simulink model "AAS"  (R2022b)
settings: Solver=ode4  StartTime=0.0  StopTime=inf  FixedStep=0.01  RelTol=1e-3  EnableMultiTasking=on
libraries: fuzblock x1
settings Model: Creator=marwa  LastModifiedBy=marwa
settings SolverCC: AlgebraicLoopSolver=TrustRegion  AutoInsertRateTranBlk=on
settings DataIOCC: LimitDataPoints=on
settings OptimizationCC: LifeSpan=inf
settings DebuggingCC: UnconnectedInputMsg=warning  UnconnectedOutputMsg=warning  UnconnectedLineMsg=warning  AllowSymbolicDim=off  SFUnexpectedBacktrackingDiag=warning  SFNoUnconditionalDefaultTransitionDiag=warning  SFExecutionAtInitializationDiag=none  ArithmeticOperatorsInVariantConditions=warning
settings ModelReferenceCC: EnableRefExpFcnMdlSchedulingChecks=on
settings SFSimCC: SimUseLocalCustomCode=off  CustomCodeUndefinedFunction=UseInterfaceOnly
settings RTWCC: RTWUseLocalCustomCode=off  DLArmComputeVersion=19.05
settings CodeAppCC: StateflowObjectComments=on
settings GRTTargetCC: TargetLangStandard=C89/C90 (ANSI)
settings ConfigComp: CovMetricSettings=dw  CovSaveCumulativeToWorkspaceVar=on  CovSaveSingleToWorkspaceVar=on  CovExternalEMLEnable=off  CovSFcnEnable=off

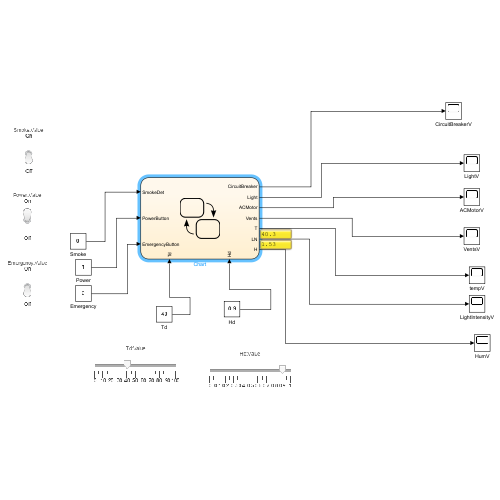
[thumbnail: Simulink's stored preview of the top-level diagram]
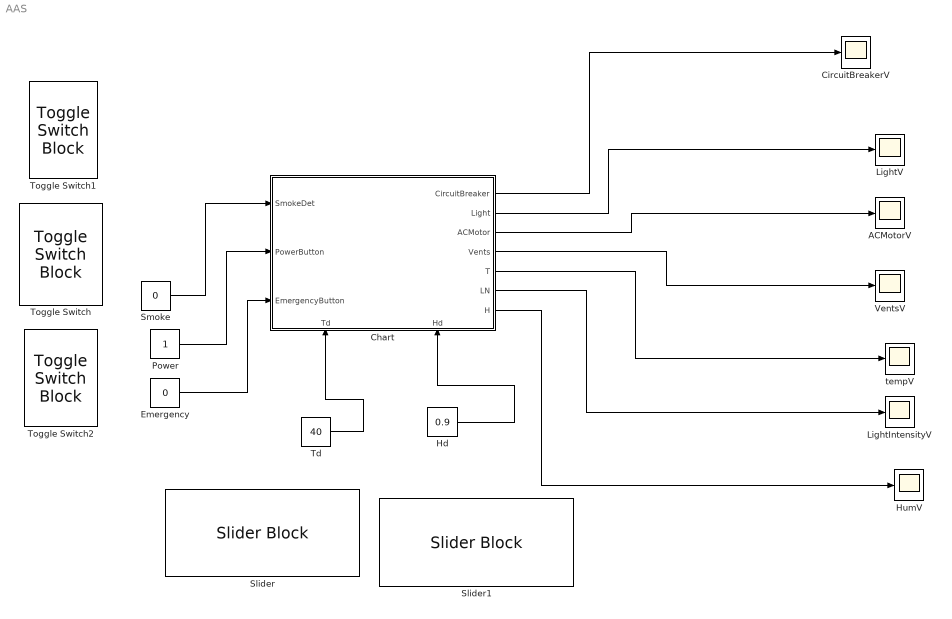
== system AAS ==
  ACMotorV : Scope
  Chart : Stateflow chart  TreatAsAtomicUnit=on
      settings: PortSchema="{\"entries\":[{\"content\":{\"sides\":[{\"content\":{\"connectorIds\":[\"In1\",\"In2\",\"In3\"]},\"type\":\"ConnectorPlacement.EquallySpacedRectSide\",\"uuid\":\"5cb868e6-5551-4fae-9f9a-b14f0c4a41d3\"},{\"content\":{\"connectorIds\":[\"Out1\",\"Out2\",\"Out3\",\"Out4\",\"Out6\",\"Out5\",\"Out7\"],\"side\":\"RIGHT\"},\"type\":\"ConnectorPlacement.EquallySpacedRectSide\",\"uuid\":\"822cf98d-9f25-4796-a860-f61431df4421\"},{\"content\":{\"connectorIds\":[],\"side\":\"TOP\"},\"type\":\"ConnectorPlacement.EquallySpacedRectSide\",\"uuid\":\"1de60880-a042-4c2a-a744-54787d460a6d\"},{\"content\":{\"connectorIds\":[\"In4\",\"In5\"],\"side\":\"BOTTOM\"},\"type\":\"ConnectorPlacement.EquallySpacedRectSide\",\"uuid\":\"160f7fd3-c7f7-4859-8f15-e416a90d14eb\"}]},\"type\":\"ConnectorPlacement.EquallySpacedConnector\",\"uuid\":\"910f53eb-049d-4d7c-afd0-ebd92eccdf07\"}],\"packageUris\":[\"http://schema.mathworks.com/mf0/Connector/R2020b\"],\"version\":\"1.0\"}"
  CircuitBreakerV : Scope
  Emergency : Constant  Value=0
  Hd : Constant  Value=0.9
  HumV : Scope
  LightIntensityV : Scope
  LightV : Scope
  Power : Constant
  Slider : SliderBlock
  Slider1 : SliderBlock  ScaleMax=1
  Smoke : Constant  Value=0
  Td : Constant  Value=40
  Toggle Switch : ToggleSwitchBlock
      settings: Values={{'Off', 'On'}, [0 1]}
  Toggle Switch1 : ToggleSwitchBlock
      settings: Values={{'Off', 'On'}, [0 1]}
  Toggle Switch2 : ToggleSwitchBlock
      settings: Values={{'Off', 'On'}, [0 1]}
  VentsV : Scope
  tempV : Scope
  wires:
  Power/1 -> Chart/2(PowerButton)
  Smoke/1 -> Chart/1(SmokeDet)
  Emergency/1 -> Chart/3(EmergencyButton)
  Chart/1(CircuitBreaker) -> CircuitBreakerV/1
  Chart/2(Light) -> LightV/1
  Chart/3(ACMotor) -> ACMotorV/1
  Chart/6(T) -> tempV/1
  Chart/4(Vents) -> VentsV/1
  Chart/5(LN) -> LightIntensityV/1
  Chart/7(H) -> HumV/1
  Td/1 -> Chart/4(Td)
  Hd/1 -> Chart/5(Hd)

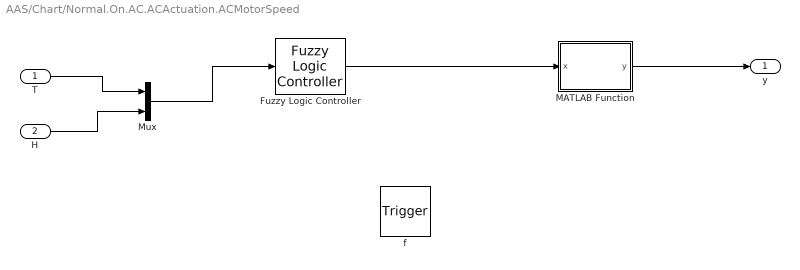
== system AAS/Chart/Normal.On.AC.ACActuation.ACMotorSpeed ==
  T : Inport  OutDataTypeStr=double  PortDimensions=1
  H : Inport  Port=2  OutDataTypeStr=double  PortDimensions=1
  f : TriggerPort  TriggerType=function-call  VariantControl=(inherit)
      settings: CopyFcn=Stateflow.SLINSF.SimulinkMan.removeBlockPreDeleteFcn  PreDeleteFcn=Stateflow.SLINSF.SimulinkMan.unsafePredeleteFcn
  Fuzzy Logic Controller : fuzblock/Fuzzy Logic  Controller  FIS=FuzzyAdvanced  OutputSampleNumber=101  DataType=double  FuzzifiedInputs=off  RuleFiringStrengths=off  RuleOutputs=off  AggregatedOutputs=off  SimulateUsing=Interpreted execution  OutOfRangeInputValueMessage=warning  NoRuleFiredMessage=warning  EmptyOutputFuzzySetMessage=warning
  MATLAB Function : MATLAB Function  TreatAsAtomicUnit=on
  Mux : Mux  Inputs=2
  y : Outport
  wires:
  T/1 -> Mux/1
  H/1 -> Mux/2
  MATLAB Function/1(y) -> y/1
  Fuzzy Logic Controller/1 -> MATLAB Function/1(x)
  Mux/1 -> Fuzzy Logic Controller/1

== matlab function AAS/Chart/Normal.On.AC.ACActuation.ACMotorSpeed/MATLAB Function ==
  data: x input; y output
function y = fcn(x)
y = 1725*(1-x)+1725;

== stateflow chart AAS/Chart ==
  settings: updateMethod=CONTINUOUS
  state Normal
    entry:
    Vents = 0;
    CircuitBreaker = 0;
    state On
      state Light [parallel]
        settings: executionOrder=2
        state LightSensing [parallel]
          settings: executionOrder=2
          state Day
            du:
            LN_dot = LN /100;
          state Night
            du:
            LN_dot = -LN/100;
          (default) -> Night
          Day -> Night : [LN > 100]
          Night -> Day : [LN < 1]
        state LightActuation [parallel]
          settings: executionOrder=1
          (history)
          state Zero
            entry:
            Light = 0;
            %0 dark
            %100 light
          state Quarter
            entry:
            Light = 25;
          state Half
            entry:
            Light = 50;
          state Maximum
            entry:
            Light = 100;
          state ThreeQuarter
            entry:
            Light = 75;
          (default) -> Zero
          Quarter -> Half [order 1] : [LN < 75]
          Zero -> Quarter : [LN < 100]
          Quarter -> Zero [order 2] : [LN >= 100]
          Half -> Quarter [order 2] : [LN >= 75]
          ThreeQuarter -> Half [order 2] : [LN >= 50]
          Half -> ThreeQuarter [order 1] : [LN < 50]
          ThreeQuarter -> Maximum [order 1] : [LN < 25]
          Maximum -> ThreeQuarter : [LN >= 25]
      state AC [parallel]
        settings: executionOrder=1
        state TempSensing [parallel]
          settings: executionOrder=1
          state Below
            du:
            T_dot = -T;
          state Over
            du:
            T_dot = 100 - T;
          state Regulated
            du:
            T_dot = 0;
          (default) -> Normal.On.AC.TempSensing.Below
          Normal.On.AC.TempSensing.Over -> Normal.On.AC.TempSensing.Below [order 1] : [int_num(T) > int_num(Td)]
          Normal.On.AC.TempSensing.Below -> Normal.On.AC.TempSensing.Over [order 1] : [int_num(T) < int_num(Td)]
          Normal.On.AC.TempSensing.Below -> Normal.On.AC.TempSensing.Regulated [order 2] : [(int_num(T) - int_num(Td) == 0) && (-T < 0) && (100 - T > 0)]
          Normal.On.AC.TempSensing.Regulated -> Normal.On.AC.TempSensing.Below [order 1] : [int_num(T) > int_num(Td)]
          Normal.On.AC.TempSensing.Over -> Normal.On.AC.TempSensing.Regulated [order 2] : [(int_num(T) - int_num(Td) == 0) && (-T < 0) && (100 - T > 0)]
          Normal.On.AC.TempSensing.Regulated -> Normal.On.AC.TempSensing.Over [order 2] : [int_num(T) < int_num(Td)]
        state ACActuation [parallel]
          du:
          ACMotor = ACMotorSpeed(T,H);
          settings: executionOrder=2
          state y = ACMotorSpeed(T,H) [function]
        state HumSensing [parallel]
          settings: executionOrder=3
          state Below
            du:
            H_dot = -H;
          state Over
            du:
            H_dot = 1 - H;
          state Regulated
            du:
            H_dot = 0;
          (default) -> Normal.On.AC.HumSensing.Below
          Normal.On.AC.HumSensing.Over -> Normal.On.AC.HumSensing.Below [order 1] : [dec_num(H) > dec_num(Hd)]
          Normal.On.AC.HumSensing.Below -> Normal.On.AC.HumSensing.Over [order 1] : [dec_num(H) < dec_num(Hd)]
          Normal.On.AC.HumSensing.Below -> Normal.On.AC.HumSensing.Regulated [order 2] : [(dec_num(H) - dec_num(Hd) == 0) && (-H < 0) && (1 - T > 0)]
          Normal.On.AC.HumSensing.Regulated -> Normal.On.AC.HumSensing.Below [order 1] : [dec_num(H) > dec_num(Hd)]
          Normal.On.AC.HumSensing.Over -> Normal.On.AC.HumSensing.Regulated [order 2] : [(dec_num(H) - dec_num(Hd) == 0) && (-H < 0) && (1 - H > 0)]
          Normal.On.AC.HumSensing.Regulated -> Normal.On.AC.HumSensing.Over [order 2] : [dec_num(H) < dec_num(Hd)]
    state Off
      entry:
      Light = 0;
      ACMotor = 0;
      CircuitBreaker = 0;
      Vents = 0;
    (default) -> Off
    Off -> On : [PowerButton == 1]
    On -> Off : [PowerButton == 0]
  state Emergency
    entry:
    Vents = 1;
    CircuitBreaker = 1;
    Light = 100;
    ACMotor = 0;
  (default) -> Normal
  Normal -> Emergency : [EmergencyButton == 1 || SmokeDet == 1]
  Emergency -> Normal : [EmergencyButton == 0 && SmokeDet == 0]
  data: Tin function_input; Tout function_output; y function_output; T function_input double size=1; H function_input double size=1; Hin function_input; Hout function_output; CircuitBreaker output; Light output; ACMotor output; Vents output; SmokeDet input; PowerButton input; EmergencyButton input; LN output =65; T output =25; Td input; H output =0.9; Hd input
  data LN settings: updateMethod=SF_CONTINUOUS_TIME_DATA
  data T settings: updateMethod=SF_CONTINUOUS_TIME_DATA
  data H settings: updateMethod=SF_CONTINUOUS_TIME_DATA
  function Tout = int_num(Tin):
    | function Tout = int_num(Tin)
    | Tout = floor(Tin);
    | end
  function Hout = dec_num(Hin):
    | function Hout = dec_num(Hin)
    | Hout = floor(Hin*100)/100;
    | end
